simulink model "QArm_Test_2"  (R2021a)
settings: Solver=ode4  StartTime=0.0  StopTime=inf  FixedStep=1/500  RelTol=1e-3  EnableMultiTasking=on
InitFcn:
  | home = [0.45; 0; 0.49];
  | A = [0.45; 0; 0.49];
  | B = [ 0.35; -0.35; 0.59];
  | C = [ 0.35; -0.35; 0.39];
  | D = [ 0.35;  0.35; 0.39];
  | E = [ 0.35;  0.35; 0.59];
  | 
  | pick_high = [0.00; -0.45; 0.15];
  | pick = [0.00; -0.45; 0.03];
  | place = [0.00; 0.45; 0.15];
  | 
  | waypoints = ...
  | [B, B, C, D, D, E]' ;
undefined symbols (not defined in the file): HIL, qc_get_step_size
libraries: quarc_library x16, simulink x3
settings Model: SimulationMode=external  ExtModeTrigDuration=10000  Creator=fvranes  LastModifiedBy=mbohra
settings SolverCC: AlgebraicLoopSolver=TrustRegion  PositivePriorityOrder=on
settings DataIOCC: SaveOutput=off  SignalLogging=off  DSMLogging=off  SaveTime=off  ReturnWorkspaceOutputs=off
settings DebuggingCC: SFMachineParentedDataDiag=warning  ArithmeticOperatorsInVariantConditions=warning
settings SFSimCC: SimUseLocalCustomCode=off  CustomCodeUndefinedFunction=UseInterfaceOnly
settings RTWCC: Description=QUARC Win64 Target Using Toolchain  SystemTargetFile=quarc_win64.tlc  TemplateMakefile=quarc_default_tmf  RTWUseLocalCustomCode=off  Toolchain=QUARC win64 | nmake (64-bit Windows)  BuildConfiguration=Faster Runs
settings CodeAppCC: StateflowObjectComments=on
settings STFCustomTargetCC: TargetLangStandard=C99 (ISO)  ConcurrentExecutionCompliant=on  SystemTargetFile=quarc_win64.tlc
settings GRTTargetCC: ParMdlRefBuildCompliant=off  CompOptLevelCompliant=off  CombineOutputUpdateFcns=off  MatFileLogging=off  CPPClassGenCompliant=off  GRTInterface=on  ExtMode=on  ExtModeMexFile=quarc_comm
settings ConfigComp: CovMetricSettings=dswe

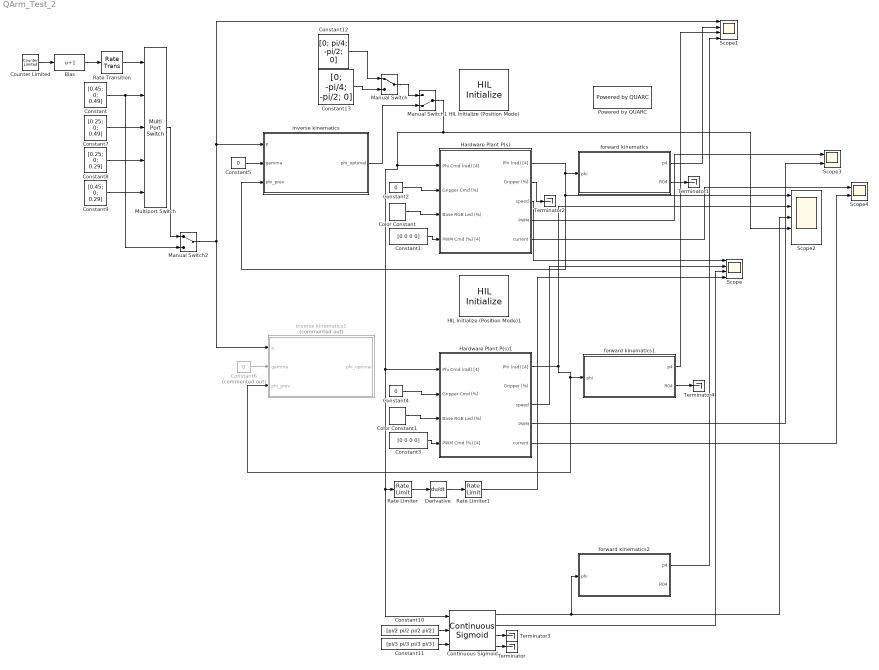
== system QArm_Test_2 ==
  Bias : Bias  Bias=1
  Color Constant : quarc_library/Sources/Signals/Color Constant  color=[0.71765 0.27451 1]
      settings: SourceProductName=QUARC Targets
  Color Constant1 : quarc_library/Sources/Signals/Color Constant  color=[0.71765 0.27451 1]
      settings: SourceProductName=QUARC Targets
  Constant : Constant  Value=[0.45; 0; 0.49]  VectorParams1D=off
  Constant1 : Constant  Value=[0 0 0 0]
  Constant10 : Constant  Value=[pi/2 pi/2 pi/2 pi/2]
  Constant11 : Constant  Value=[pi/3 pi/3 pi/3 pi/3]
  Constant12 : Constant  Value=[0; pi/4; -pi/2; 0]  VectorParams1D=off
  Constant13 : Constant  Value=[0; -pi/4; -pi/2; 0]  VectorParams1D=off
  Constant2 : Constant  Value=0
  Constant3 : Constant  Value=[0 0 0 0]
  Constant4 : Constant  Value=0
  Constant5 : Constant  Value=0
  Constant6 : Constant  Commented=on  Value=0
  Constant7 : Constant  Value=[0.25; 0; 0.49]  VectorParams1D=off
  Constant8 : Constant  Value=[0.25; 0; 0.29]  VectorParams1D=off
  Constant9 : Constant  Value=[0.45; 0; 0.29]  VectorParams1D=off
  Continuous Sigmoid : quarc_library/Sources/Sigmoids/Continuous Sigmoid  params_source=External (input ports)  max_velocity=10  max_acceleration=10  initial_position=0  initial_velocity=0  hold_off=qc_get_step_size  input_sample_time=qc_get_step_size  output_sample_time=qc_get_step_size
      settings: SourceProductName=QUARC Targets
  Counter Limited : simulink/Sources/Counter Limited  uplimit=3  tsamp=4
  Derivative : Derivative
  HIL Initialize (Position Mode) : quarc_library/Data Acquisition/Generic/Configuration/HIL Initialize  Priority=2  object_name=HIL-1  board_type=qarm_usb  board_number=0  board_options=j0_mode=0;j1_mode=0;j2_mode=0;j3_mode=0;gripper_mode=0;j0_profile_config=0;j0_profile_velocity=1.5708;j0_profile_acceleration=1.0472;j1_profile_config=0;j1_profile_velocity=1.5708;j1_profile_acceleration=1.0472;j2_profile_config=0;j2_profile_velocity=1.5708;j2_profile_acceleration=1.0472;j3_profile_config=0;j3_profile_velocity=1.5708;j3_profile_acceleration=1.0472;  exclusive=off  active=on  hardware_clocks=[0]  clock_modes=[]  initial_clock_frequencies=[]  set_clock_params_at_start=off  set_clock_params_at_switch_in=off  set_clock_frequencies_at_start=off  set_clock_frequencies_at_switch_in=off  analog_input_channels=[5:9]  analog_input_configurations=[]  analog_input_maximums=[]  analog_input_minimums=[]  set_analog_input_params_at_start=off  set_analog_input_params_at_switch_in=off  analog_output_channels=[]  analog_output_maximums=inf  analog_output_minimums=-inf  initial_analog_outputs=[0]  final_analog_outputs=[0]  watchdog_analog_outputs=[]  set_analog_output_params_at_start=off  set_analog_output_params_at_switch_in=off  set_analog_outputs_at_start=off  set_analog_outputs_at_switch_in=off  set_analog_outputs_at_terminate=off  set_analog_outputs_at_switch_out=off  set_analog_outputs_on_watchdog=off  digital_input_channels=[]  digital_output_channels=[]  digital_output_configuration=[]  initial_digital_outputs=[0]  final_digital_outputs=[0]  watchdog_digital_outputs=[0]  set_digital_output_params_at_start=off  set_digital_output_params_at_switch_in=off  set_digital_outputs_at_start=off  set_digital_outputs_at_switch_in=off  set_digital_outputs_at_terminate=off  set_digital_outputs_at_switch_out=off  set_digital_outputs_on_watchdog=off  encoder_channels=[]  quadrature=[]  encoder_filter_frequency=[]  initial_encoder_counts=[]  set_encoder_params_at_start=off  set_encoder_params_at_switch_in=off  set_encoder_counts_at_start=off  set_encoder_counts_at_switch_in=off  pwm_channels=[]  pwm_modes=[]  pwm_frequency=[]  pwm_configuration=[]  pwm_alignment=[]  pwm_polarity=[]  pwm_leading_deadband=[]  pwm_trailing_deadband=[]  initial_pwm_outputs=[]  final_pwm_outputs=[]  watchdog_pwm_outputs=[]  set_pwm_params_at_start=off  set_pwm_params_at_switch_in=off  set_pwm_outputs_at_start=off  set_pwm_outputs_at_switch_in=off  set_pwm_outputs_at_terminate=off  set_pwm_outputs_at_switch_out=off  set_pwm_outputs_on_watchdog=off  other_output_channels=[11005:11008]  initial_other_outputs=[0 1 0 1]  final_other_outputs=[1 0 0 0]  watchdog_other_outputs=[0 0 1 0]  set_other_outputs_at_start=on  set_other_outputs_at_switch_in=off  set_other_outputs_at_terminate=on  set_other_outputs_at_switch_out=off  set_other_outputs_on_watchdog=off
  HIL Initialize (Position Mode)1 : quarc_library/Data Acquisition/Generic/Configuration/HIL Initialize  Priority=2  object_name=HIL-2  board_type=qarm_usb  board_number=0@tcpip://localhost:18900  board_options=j0_mode=0;j1_mode=0;j2_mode=0;j3_mode=0;gripper_mode=0;j0_profile_config=0;j0_profile_velocity=1.5708;j0_profile_acceleration=1.0472;j1_profile_config=0;j1_profile_velocity=1.5708;j1_profile_acceleration=1.0472;j2_profile_config=0;j2_profile_velocity=1.5708;j2_profile_acceleration=1.0472;j3_profile_config=0;j3_profile_velocity=1.5708;j3_profile_acceleration=1.0472;  exclusive=off  active=on  hardware_clocks=[0]  clock_modes=[]  initial_clock_frequencies=[]  set_clock_params_at_start=off  set_clock_params_at_switch_in=off  set_clock_frequencies_at_start=off  set_clock_frequencies_at_switch_in=off  analog_input_channels=[5:9]  analog_input_configurations=[]  analog_input_maximums=[]  analog_input_minimums=[]  set_analog_input_params_at_start=off  set_analog_input_params_at_switch_in=off  analog_output_channels=[]  analog_output_maximums=inf  analog_output_minimums=-inf  initial_analog_outputs=[0]  final_analog_outputs=[0]  watchdog_analog_outputs=[]  set_analog_output_params_at_start=off  set_analog_output_params_at_switch_in=off  set_analog_outputs_at_start=off  set_analog_outputs_at_switch_in=off  set_analog_outputs_at_terminate=off  set_analog_outputs_at_switch_out=off  set_analog_outputs_on_watchdog=off  digital_input_channels=[]  digital_output_channels=[]  digital_output_configuration=[]  initial_digital_outputs=[0]  final_digital_outputs=[0]  watchdog_digital_outputs=[0]  set_digital_output_params_at_start=off  set_digital_output_params_at_switch_in=off  set_digital_outputs_at_start=off  set_digital_outputs_at_switch_in=off  set_digital_outputs_at_terminate=off  set_digital_outputs_at_switch_out=off  set_digital_outputs_on_watchdog=off  encoder_channels=[]  quadrature=[]  encoder_filter_frequency=[]  initial_encoder_counts=[]  set_encoder_params_at_start=off  set_encoder_params_at_switch_in=off  set_encoder_counts_at_start=off  set_encoder_counts_at_switch_in=off  pwm_channels=[]  pwm_modes=[]  pwm_frequency=[]  pwm_configuration=[]  pwm_alignment=[]  pwm_polarity=[]  pwm_leading_deadband=[]  pwm_trailing_deadband=[]  initial_pwm_outputs=[]  final_pwm_outputs=[]  watchdog_pwm_outputs=[]  set_pwm_params_at_start=off  set_pwm_params_at_switch_in=off  set_pwm_outputs_at_start=off  set_pwm_outputs_at_switch_in=off  set_pwm_outputs_at_terminate=off  set_pwm_outputs_at_switch_out=off  set_pwm_outputs_on_watchdog=off  other_output_channels=[11005:11008]  initial_other_outputs=[0 1 0 1]  final_other_outputs=[1 0 0 0]  watchdog_other_outputs=[0 0 1 0]  set_other_outputs_at_start=on  set_other_outputs_at_switch_in=off  set_other_outputs_at_terminate=on  set_other_outputs_at_switch_out=off  set_other_outputs_on_watchdog=off
  Hardware Plant P(s) : Subsystem
  Hardware Plant P(s)1 : Subsystem
  Manual Switch : ManualSwitch
  Manual Switch1 : ManualSwitch  CurrentSetting=0
  Manual Switch2 : ManualSwitch
  Multiport Switch : MultiPortSwitch  Inputs=4
  Powered by QUARC : quarc_library/Logos/Powered by QUARC
  Rate Limiter : RateLimiter  RisingSlewLimit=pi/2  FallingSlewLimit=-pi/2  SampleTimeMode=inherited
  Rate Limiter1 : RateLimiter  RisingSlewLimit=pi/3  FallingSlewLimit=-pi/3  SampleTimeMode=inherited
  Rate Transition : RateTransition
  Scope : Scope  NumInputPorts=4
  Scope1 : Scope  NumInputPorts=4
  Scope2 : Scope  NumInputPorts=5
  Scope3 : Scope  NumInputPorts=2
  Scope4 : Scope  NumInputPorts=2
  Terminator{,1..4} (5 alike) : Terminator
  forward kinematics : MATLAB Function  TreatAsAtomicUnit=on
  forward kinematics1 : MATLAB Function  TreatAsAtomicUnit=on
  forward kinematics2 : MATLAB Function  TreatAsAtomicUnit=on
  inverse kinematics : MATLAB Function  TreatAsAtomicUnit=on
  inverse kinematics1 : MATLAB Function  Commented=on  TreatAsAtomicUnit=on
  wires:
  Hardware Plant P(s)/2(Gripper (%)) -> Terminator2/1
  Hardware Plant P(s)/1(Phi (rad) [4]) -> inverse kinematics/3(phi_prev), Scope2/1, forward kinematics/1(phi)
  Color Constant/1 -> Hardware Plant P(s)/3(Base RGB Led (%))
  Constant1/1 -> Hardware Plant P(s)/4(PWM Cmd (%) [4])
  Constant5/1 -> inverse kinematics/2(gamma)
  Manual Switch1/1 -> Continuous Sigmoid/1, Rate Limiter/1, Hardware Plant P(s)1/1(Phi Cmd (rad) [4]), Hardware Plant P(s)/1(Phi Cmd (rad) [4]), Scope2/4
  Constant2/1 -> Hardware Plant P(s)/2(Gripper Cmd (%))
  forward kinematics/1(p4) -> Scope1/2
  forward kinematics/2(R04) -> Terminator1/1
  Constant4/1 -> Hardware Plant P(s)1/2(Gripper Cmd (%))
  Color Constant1/1 -> Hardware Plant P(s)1/3(Base RGB Led (%))
  Constant3/1 -> Hardware Plant P(s)1/4(PWM Cmd (%) [4])
  Manual Switch2/1 -> Scope1/1, inverse kinematics/1(p), inverse kinematics1/1(p)
  Constant6/1 -> inverse kinematics1/2(gamma)
  forward kinematics1/2(R04) -> Terminator4/1
  forward kinematics1/1(p4) -> Scope1/3
  Hardware Plant P(s)1/1(Phi (rad) [4]) -> inverse kinematics1/3(phi_prev), forward kinematics1/1(phi), Scope2/2
  Hardware Plant P(s)/3(speed) -> Scope/1
  Hardware Plant P(s)1/3(speed) -> Scope/2
  Constant/1 -> Manual Switch2/2, Multiport Switch/2
  Constant7/1 -> Multiport Switch/3
  Constant8/1 -> Multiport Switch/4
  Constant9/1 -> Multiport Switch/5
  Bias/1 -> Rate Transition/1
  Counter Limited/1 -> Bias/1
  Rate Transition/1 -> Multiport Switch/1
  Continuous Sigmoid/3 -> Terminator3/1
  Continuous Sigmoid/4 -> Terminator/1
  Constant11/1 -> Continuous Sigmoid/3
  Constant10/1 -> Continuous Sigmoid/2
  Continuous Sigmoid/1 -> forward kinematics2/1(phi), Scope2/3
  Continuous Sigmoid/2 -> Scope/3
  forward kinematics2/1(p4) -> Scope1/4
  Constant13/1 -> Manual Switch/2
  Constant12/1 -> Manual Switch/1
  Manual Switch/1 -> Manual Switch1/1
  inverse kinematics/1(phi_optimal) -> Manual Switch1/2
  Multiport Switch/1 -> Manual Switch2/1
  Rate Limiter/1 -> Derivative/1
  Derivative/1 -> Rate Limiter1/1
  Rate Limiter1/1 -> Scope/4
  Hardware Plant P(s)/4(PWM) -> Scope3/1
  Hardware Plant P(s)1/4(PWM) -> Scope3/2
  Hardware Plant P(s)/5(current) -> Scope4/1
  Hardware Plant P(s)1/5(current) -> Scope4/2

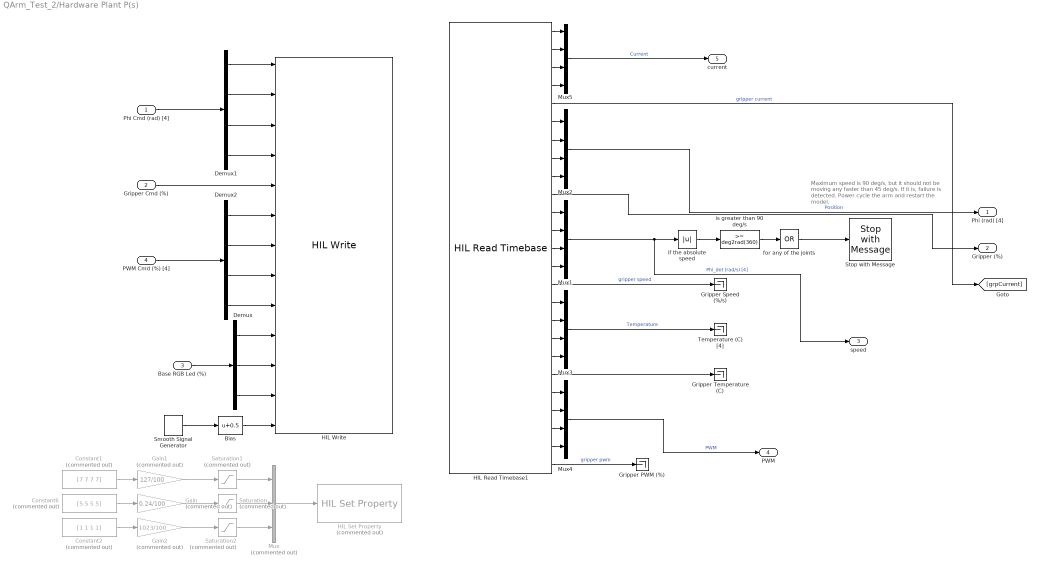
== system QArm_Test_2/Hardware Plant P(s) ==
  note: Maximum speed is 90 deg/s, but it should not
      | be moving any faster than 45 deg/s. If it is,
      | failure is detected. Power cycle the arm and
      | restart the model.
  Phi Cmd (rad) [4] : Inport
  Gripper Cmd (%) : Inport  Port=2
  Base RGB Led (%) : Inport  Port=3
  PWM Cmd (%) [4] : Inport  Port=4
  Bias : Bias  Bias=0.5
  Constant1 : Constant  Commented=on  Value=[7 7 7 7]
  Constant2 : Constant  Commented=on  Value=[1 1 1 1]
  Constant6 : Constant  Commented=on  Value=[5 5 5 5]
  Demux : Demux  Outputs=3
  Demux1 : Demux
  Demux2 : Demux
  Gain : Gain  Commented=on  Gain=0.24/100
  Gain1 : Gain  Commented=on  Gain=127/100
  Gain2 : Gain  Commented=on  Gain=1023/100
  Gripper PWM (%) : Terminator
  Gripper Speed (%/s) : Terminator
  Gripper Temperature (C) : Terminator
  HIL Read Timebase1 : quarc_library/Data Acquisition/Generic/Timebases/HIL Read Timebase  object_name=HIL-1  clock=0  analog_channels=[5:9]  encoder_channels=[]  digital_channels=[]  other_channels=[1000:1004 3000:3004 10000:10004 11000:11004]  active=on  vector_output=off  data_type_mode=Inherit via back propagation  encoder_data_type=double  digital_data_type=boolean  overflow_mode=Error on overflow  samples_in_buffer=max(ceil(1/qc_get_step_size), 1)
  HIL Set Property : quarc_library/Data Acquisition/Generic/Configuration/HIL Set Property  Commented=on  object_name=HIL-1  property_type=2  property_codes=[128:131, 133:136, 138:141]  property_source=2  property_value_num=0  set_at_start=on  sample_time=-1  active=off
      settings: AttributesFormatString=(%<object_name>)  SourceProductName=QUARC Targets
  HIL Write : quarc_library/Data Acquisition/Generic/Immediate I//O/HIL Write  object_name=HIL-1  analog_channels=[]  pwm_channels=[]  digital_channels=[]  other_channels=[1000:1004 11000:11003 11005:11008]  sample_time=-1  active=on  vector_input=off
  Mux : Mux  Commented=on  Inputs=3
  Mux{1..5} (5 alike) : Mux
  Saturation : Saturate  Commented=on  UpperLimit=0.24  LowerLimit=0
  Saturation1 : Saturate  Commented=on  UpperLimit=127  LowerLimit=0
  Saturation2 : Saturate  Commented=on  UpperLimit=1023  LowerLimit=0
  Smooth Signal Generator : quarc_library/Sources/Signals/Smooth Signal Generator  signal_type=Sine  source=Internal (dialog parameters)  amplitude=0.5  frequency=0.5  initial_phase=0  sample_time=qc_get_step_size  output_cos=off
      settings: SourceProductName=QUARC Targets
  Stop with Message : quarc_library/Sinks/Error Handling/Stop with Message  message_type=Fixed error message  message_icon=Error  message=Arm moving close to maximum speed.
  Temperature (C) [4] : Terminator
  for any of the joints : Logic  Operator=OR  Inputs=1  IconShape=distinctive  AllPortsSameDT=off  OutDataTypeStr=boolean
  if the absolute speed : Abs
  is greater than 90 deg/s : simulink/Logic and Bit Operations/Compare To Constant  relop=>=  const=deg2rad(360)  OutDataTypeStr=boolean
  Phi (rad) [4] : Outport  VectorParamsAs1DForOutWhenUnconnected=off
  Gripper (%) : Outport  Port=2  VectorParamsAs1DForOutWhenUnconnected=off
  speed : Outport  Port=3  VectorParamsAs1DForOutWhenUnconnected=off
  PWM : Outport  Port=4  VectorParamsAs1DForOutWhenUnconnected=off
  current : Outport  Port=5  VectorParamsAs1DForOutWhenUnconnected=off
  wires:
  HIL Read Timebase1/10 -> Gripper (%)/1
  Constant6/1 -> Gain/1
  Saturation/1 -> Mux/2
  Gain/1 -> Saturation/1
  Mux/1 -> HIL Set Property/1
  Gain1/1 -> Saturation1/1
  Constant1/1 -> Gain1/1
  Constant2/1 -> Gain2/1
  Gain2/1 -> Saturation2/1
  Saturation2/1 -> Mux/3
  Saturation1/1 -> Mux/1
  Demux1/4 -> HIL Write/4
  Base RGB Led (%)/1 -> Demux/1
  Demux/2 -> HIL Write/11
  Demux/1 -> HIL Write/10
  Demux1/2 -> HIL Write/2
  Gripper Cmd (%)/1 -> HIL Write/5
  Bias/1 -> HIL Write/13
  Phi Cmd (rad) [4]/1 -> Demux1/1
  Smooth Signal Generator/1 -> Bias/1
  Demux/3 -> HIL Write/12
  Demux1/3 -> HIL Write/3
  PWM Cmd (%) [4]/1 -> Demux2/1
  Demux2/2 -> HIL Write/7
  Demux2/1 -> HIL Write/6
  Demux1/1 -> HIL Write/1
  Demux2/4 -> HIL Write/9
  Demux2/3 -> HIL Write/8
  for any of the joints/1 -> Stop with Message/1
  is greater than 90 deg/s/1 -> for any of the joints/1
  if the absolute speed/1 -> is greater than 90 deg/s/1
  HIL Read Timebase1/16 -> Mux3/1
  HIL Read Timebase1/12 -> Mux1/2
  HIL Read Timebase1/4 -> Mux5/4
  HIL Read Timebase1/5 -> [grpCurrent]  "gripper current"
  HIL Read Timebase1/11 -> Mux1/1
  HIL Read Timebase1/14 -> Mux1/4
  HIL Read Timebase1/6 -> Mux2/1
  HIL Read Timebase1/19 -> Mux3/4
  HIL Read Timebase1/8 -> Mux2/3
  Mux5/1 -> current/1  "Current"
  HIL Read Timebase1/7 -> Mux2/2
  HIL Read Timebase1/24 -> Mux4/4
  HIL Read Timebase1/1 -> Mux5/1
  HIL Read Timebase1/2 -> Mux5/2
  HIL Read Timebase1/21 -> Mux4/1
  HIL Read Timebase1/20 -> Gripper Temperature (C)/1
  HIL Read Timebase1/22 -> Mux4/2
  HIL Read Timebase1/17 -> Mux3/2
  HIL Read Timebase1/18 -> Mux3/3
  Mux4/1 -> PWM/1  "PWM"
  HIL Read Timebase1/13 -> Mux1/3
  HIL Read Timebase1/23 -> Mux4/3
  HIL Read Timebase1/3 -> Mux5/3
  HIL Read Timebase1/25 -> Gripper PWM (%)/1  "gripper pwm"
  Mux3/1 -> Temperature (C) [4]/1  "Temperature"
  HIL Read Timebase1/9 -> Mux2/4
  Mux2/1 -> Phi (rad) [4]/1  "Position"
  Mux1/1 -> speed/1, if the absolute speed/1  "Phi_dot (rad/s) [4]"
  HIL Read Timebase1/15 -> Gripper Speed (%/s)/1  "gripper speed"

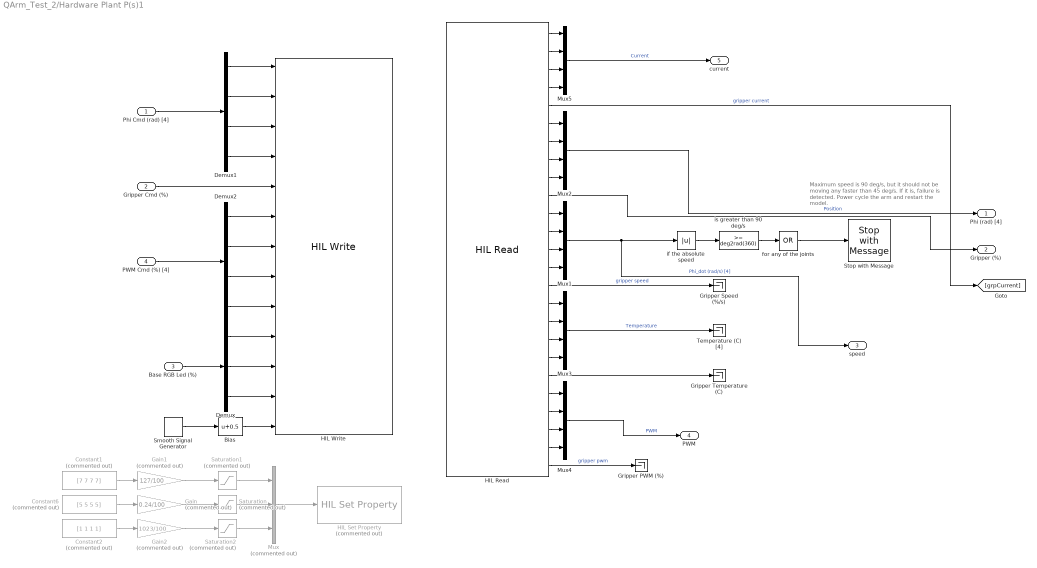
== system QArm_Test_2/Hardware Plant P(s)1 ==
  note: Maximum speed is 90 deg/s, but it should not
      | be moving any faster than 45 deg/s. If it is,
      | failure is detected. Power cycle the arm and
      | restart the model.
  Phi Cmd (rad) [4] : Inport
  Gripper Cmd (%) : Inport  Port=2
  Base RGB Led (%) : Inport  Port=3
  PWM Cmd (%) [4] : Inport  Port=4
  Bias : Bias  Bias=0.5
  Constant1 : Constant  Commented=on  Value=[7 7 7 7]
  Constant2 : Constant  Commented=on  Value=[1 1 1 1]
  Constant6 : Constant  Commented=on  Value=[5 5 5 5]
  Demux : Demux  Outputs=3
  Demux1 : Demux
  Demux2 : Demux
  Gain : Gain  Commented=on  Gain=0.24/100
  Gain1 : Gain  Commented=on  Gain=127/100
  Gain2 : Gain  Commented=on  Gain=1023/100
  Gripper PWM (%) : Terminator
  Gripper Speed (%/s) : Terminator
  Gripper Temperature (C) : Terminator
  HIL Read : quarc_library/Data Acquisition/Generic/Immediate I//O/HIL Read  object_name=HIL-2  analog_channels=[5:9]  encoder_channels=[]  digital_channels=[]  other_channels=[1000:1004 3000:3004 10000:10004 11000:11004]  sample_time=qc_get_step_size  active=on  vector_output=off  data_type_mode=Inherit via back propagation  encoder_data_type=double  digital_data_type=boolean
  HIL Set Property : quarc_library/Data Acquisition/Generic/Configuration/HIL Set Property  Commented=on  object_name=HIL-2  property_type=2  property_codes=[128:131, 133:136, 138:141]  property_source=2  property_value_num=0  set_at_start=on  sample_time=-1  active=off
      settings: AttributesFormatString=(%<object_name>)  SourceProductName=QUARC Targets
  HIL Write : quarc_library/Data Acquisition/Generic/Immediate I//O/HIL Write  object_name=HIL-2  analog_channels=[]  pwm_channels=[]  digital_channels=[]  other_channels=[1000:1004 11000:11003 11005:11008]  sample_time=-1  active=on  vector_input=off
  Mux : Mux  Commented=on  Inputs=3
  Mux{1..5} (5 alike) : Mux
  Saturation : Saturate  Commented=on  UpperLimit=0.24  LowerLimit=0
  Saturation1 : Saturate  Commented=on  UpperLimit=127  LowerLimit=0
  Saturation2 : Saturate  Commented=on  UpperLimit=1023  LowerLimit=0
  Smooth Signal Generator : quarc_library/Sources/Signals/Smooth Signal Generator  signal_type=Sine  source=Internal (dialog parameters)  amplitude=0.5  frequency=0.5  initial_phase=0  sample_time=qc_get_step_size  output_cos=off
      settings: SourceProductName=QUARC Targets
  Stop with Message : quarc_library/Sinks/Error Handling/Stop with Message  message_type=Fixed error message  message_icon=Error  message=Arm moving close to maximum speed.
  Temperature (C) [4] : Terminator
  for any of the joints : Logic  Operator=OR  Inputs=1  IconShape=distinctive  AllPortsSameDT=off  OutDataTypeStr=boolean
  if the absolute speed : Abs
  is greater than 90 deg/s : simulink/Logic and Bit Operations/Compare To Constant  relop=>=  const=deg2rad(360)  OutDataTypeStr=boolean
  Phi (rad) [4] : Outport  VectorParamsAs1DForOutWhenUnconnected=off
  Gripper (%) : Outport  Port=2  VectorParamsAs1DForOutWhenUnconnected=off
  speed : Outport  Port=3  VectorParamsAs1DForOutWhenUnconnected=off
  PWM : Outport  Port=4  VectorParamsAs1DForOutWhenUnconnected=off
  current : Outport  Port=5  VectorParamsAs1DForOutWhenUnconnected=off
  wires:
  HIL Read/15 -> Gripper Speed (%/s)/1  "gripper speed"
  Mux2/1 -> Phi (rad) [4]/1  "Position"
  HIL Read/9 -> Mux2/4
  Mux3/1 -> Temperature (C) [4]/1  "Temperature"
  HIL Read/25 -> Gripper PWM (%)/1  "gripper pwm"
  HIL Read/3 -> Mux5/3
  HIL Read/23 -> Mux4/3
  HIL Read/13 -> Mux1/3
  Mux4/1 -> PWM/1  "PWM"
  HIL Read/18 -> Mux3/3
  HIL Read/17 -> Mux3/2
  HIL Read/22 -> Mux4/2
  HIL Read/20 -> Gripper Temperature (C)/1
  HIL Read/21 -> Mux4/1
  HIL Read/2 -> Mux5/2
  HIL Read/1 -> Mux5/1
  HIL Read/24 -> Mux4/4
  HIL Read/7 -> Mux2/2
  Mux5/1 -> current/1  "Current"
  HIL Read/8 -> Mux2/3
  HIL Read/19 -> Mux3/4
  HIL Read/6 -> Mux2/1
  HIL Read/14 -> Mux1/4
  HIL Read/11 -> Mux1/1
  HIL Read/5 -> [grpCurrent]  "gripper current"
  HIL Read/4 -> Mux5/4
  HIL Read/12 -> Mux1/2
  HIL Read/16 -> Mux3/1
  if the absolute speed/1 -> is greater than 90 deg/s/1
  is greater than 90 deg/s/1 -> for any of the joints/1
  for any of the joints/1 -> Stop with Message/1
  Demux2/3 -> HIL Write/8
  Demux2/4 -> HIL Write/9
  Demux1/1 -> HIL Write/1
  Demux2/1 -> HIL Write/6
  Demux2/2 -> HIL Write/7
  PWM Cmd (%) [4]/1 -> Demux2/1
  Demux1/3 -> HIL Write/3
  Demux/3 -> HIL Write/12
  Smooth Signal Generator/1 -> Bias/1
  Phi Cmd (rad) [4]/1 -> Demux1/1
  Bias/1 -> HIL Write/13
  Gripper Cmd (%)/1 -> HIL Write/5
  Demux1/2 -> HIL Write/2
  Demux/1 -> HIL Write/10
  Demux/2 -> HIL Write/11
  Base RGB Led (%)/1 -> Demux/1
  Demux1/4 -> HIL Write/4
  Saturation1/1 -> Mux/1
  Saturation2/1 -> Mux/3
  Gain2/1 -> Saturation2/1
  Constant2/1 -> Gain2/1
  Constant1/1 -> Gain1/1
  Gain1/1 -> Saturation1/1
  Mux/1 -> HIL Set Property/1
  Gain/1 -> Saturation/1
  Saturation/1 -> Mux/2
  Constant6/1 -> Gain/1
  HIL Read/10 -> Gripper (%)/1
  Mux1/1 -> speed/1, if the absolute speed/1  "Phi_dot (rad/s) [4]"

== matlab function QArm_Test_2/inverse kinematics1 ==
  data: p input; gamma input; phi_optimal output; phi_prev input
function phi_optimal = qarmInverseKinematics(p, gamma, phi_prev)

%% QUANSER_ARM_IPK
% v 4.0 - 4th June 2020

% REFERENCE: 
% Chapter 4. Inverse Kinematics
% Robot Dynamics and Control 
% Spong, Vidyasagar
% 1989

% INPUTS:
% p        : end-effector position vector expressed in base frame {0}
% gamma    : wrist rotation angle gamma

% OUTPUTS:
% phi_optimal : Best solution depending on phi_prev
% phi         : All four Inverse Kinematics solutions as a 4x4 matrix. 
%               Each col is a solution.

%% Manipulator parameters:
L1 = 0.1400;
L2 = 0.3500;
L3 = 0.0500;
L4 = 0.2500;
L5 = 0.1500;
beta = atan(L3/L2);

%% Alternate parameters
lambda1 = L1;
lambda2 = sqrt(L2^2 + L3^2);
lambda3 = L4 + L5;

%% Initialization
theta   = zeros(4, 4);
phi = zeros(4, 4);

%% Joint angle 2 and 3: 
% Equations:
    % lambda2 cos(theta2) + (-lambda3) sin(theta2 + theta3) = sqrt(x^2 + y^2)
    %   A     cos( 2    ) +     C      sin(   2   +    3  ) =    D
    
    % lambda2 sin(theta2) - (-lambda3) cos(theta2 + theta3) = lambda1 - z
    %   A     sin( 2    ) -     C      cos(   2   +    3  ) =    H

% Solution:
    A = lambda2;
    C = -lambda3;
    H =  lambda1 - p(3);
    D1 = -sqrt(p(1)^2 + p(2)^2);
    D2 = sqrt(p(1)^2 + p(2)^2);
    F = (D1^2 + H^2 - A^2 - C^2)/(2*A);

    theta(3,1) = 2*atan2( C + sqrt(C^2 - F^2) , F );
	theta(3,2) = 2*atan2( C - sqrt(C^2 - F^2) , F );
    theta(3,3) = 2*atan2( C + sqrt(C^2 - F^2) , F );
	theta(3,4) = 2*atan2( C - sqrt(C^2 - F^2) , F );

    M = A + C*sin(theta(3,1));
    N = -C*cos(theta(3,1));
    cos_term = (D1*M + H*N)/(M^2 + N^2);
    sin_term = (H - N*cos_term)/(M);
    theta(2,1) = atan2(sin_term, cos_term);

    M = A + C*sin(theta(3,2));
    N = -C*cos(theta(3,2));
    cos_term = (D1*M + H*N)/(M^2 + N^2);
    sin_term = (H - N*cos_term)/(M);
    theta(2,2) = atan2(sin_term, cos_term);

    M = A + C*sin(theta(3,3));
    N = -C*cos(theta(3,3));
    cos_term = (D2*M + H*N)/(M^2 + N^2);
    sin_term = (H - N*cos_term)/(M);
    theta(2,3) = atan2(sin_term, cos_term);

    M = A + C*sin(theta(3,4));
    N = -C*cos(theta(3,4));
    cos_term = (D2*M + H*N)/(M^2 + N^2);
    sin_term = (H - N*cos_term)/(M);
    theta(2,4) = atan2(sin_term, cos_term);


%% Joint angle 1:
% Equation:
    % y / x = tan(theta1);

% Solution
    theta(1,1) = atan2( p(2)/( lambda2 * cos( theta(2,1) ) - lambda3 * sin( theta(2,1) + theta(3,1) ) ) , p(1)/(  lambda2 * cos( theta(2,1) ) - lambda3 * sin( theta(2,1) + theta(3,1) )  ) );
    theta(1,2) = atan2( p(2)/( lambda2 * cos( theta(2,2) ) - lambda3 * sin( theta(2,2) + theta(3,2) ) ) , p(1)/(  lambda2 * cos( theta(2,2) ) - lambda3 * sin( theta(2,2) + theta(3,2) )  ) );
    theta(1,3) = atan2( p(2)/( lambda2 * cos( theta(2,3) ) - lambda3 * sin( theta(2,3) + theta(3,3) ) ) , p(1)/(  lambda2 * cos( theta(2,3) ) - lambda3 * sin( theta(2,3) + theta(3,3) )  ) );
    theta(1,4) = atan2( p(2)/( lambda2 * cos( theta(2,4) ) - lambda3 * sin( theta(2,4) + theta(3,4) ) ) , p(1)/(  lambda2 * cos( theta(2,4) ) - lambda3 * sin( theta(2,4) + theta(3,4) )  ) );
    
%% Remap theta back to phi
% phi(1) = theta(1);
% phi(2) = theta(2) - beta + pi/2;
% phi(3) = theta(3) + beta;
% phi(4) = theta(4);

phi(1,:) = theta(1,:);
phi(2,:) = theta(2,:) - beta + pi/2;
phi(3,:) = theta(3,:) + beta;
phi(4,:) = gamma;

phi = mod(phi + pi, 2*pi) - pi;

phi_optimal = phi(:,1);
if (norm(phi_optimal - phi_prev) > norm(phi(:,2) - phi_prev)) || (check_joint_limits(phi_optimal))
    phi_optimal = phi(:,2);
end
if (norm(phi_optimal - phi_prev) > norm(phi(:,3) - phi_prev)) || (check_joint_limits(phi_optimal))
    phi_optimal = phi(:,3);
end
if (norm(phi_optimal - phi_prev) > norm(phi(:,4) - phi_prev)) || (check_joint_limits(phi_optimal))
    phi_optimal = phi(:,4);
end
if (check_joint_limits(phi_optimal))
    phi_optimal = [0;0;0;0];
end

end

function flag = check_joint_limits(phi)
    flag = 0;
    if phi(1) > 170*pi/180 || phi(1) < -170*pi/180 ...
        || phi(2) > 80*pi/180 || phi(2) < -80*pi/180 ...
        || phi(3) > 75*pi/180 || phi(3) < -95*pi/180 ...
        || phi(4) > 160*pi/180 || phi(4) < -160*pi/180
    flag = 1;
    end
end

== matlab function QArm_Test_2/forward kinematics1 ==
  data: phi input; p4 output; R04 output
function [p4, R04] = qarmForwardKinematics(phi)

%% QUANSER_ARM_FPK
% v 4.0 - 4th June 2020

% REFERENCE: 
% Chapter 3. Forward Kinematics
% Robot Dynamics and Control 
% Spong, Vidyasagar
% 1989

% INPUTS:
% phi     : Alternate joint angles vector 4 x 1

% OUTPUTS:
% p4      : End-effector frame {4} position vector expressed in base frame {0}
% R04     : rotation matrix from end-effector frame {4} to base frame {0}

%% Manipulator parameters:
L1 = 0.1400;
L2 = 0.3500;
L3 = 0.0500;
L4 = 0.2500;
L5 = 0.1500;

%% Alternate parameters
l1 = L1;
l2 = sqrt(L2^2 + L3^2);
l3 = L4 + L5;
beta = atan(L3/L2);

%% From phi space to theta space 
theta = phi;
theta(1) = phi(1);
theta(2) = phi(2) + beta - pi/2;
theta(3) = phi(3) - beta;
theta(4) = phi(4);

%% Transformation matrices for all frames:

% T{i-1}{i} = quanser_arm_DH(  a, alpha,  d,     theta );
        T01 = quanser_arm_DH(  0, -pi/2, l1,  theta(1) );
        T12 = quanser_arm_DH( l2,     0,  0,  theta(2) );
        T23 = quanser_arm_DH(  0, -pi/2,  0,  theta(3) );
        T34 = quanser_arm_DH(  0,     0, l3,  theta(4) );

        T02 = T01*T12;
        T03 = T02*T23;
        T04 = T03*T34;

%% Position of end-effector Transformation

% Extract the Position vector 
% p1   = T01(1:3,4);
% p2   = T02(1:3,4);
% p3   = T03(1:3,4);
p4   = T04(1:3,4);

% Extract the Rotation matrix
% R01 = T01(1:3,1:3);
% R02 = T02(1:3,1:3);
% R03 = T03(1:3,1:3);
R04 = T04(1:3,1:3);

end

function T = quanser_arm_DH(a,alpha,d,theta)

%% QUANSER_ARM_DH
% v 1.0 - 26th March 2019

% REFERENCE: 
% Chapter 3. Forward and Inverse Kinematics
% Robot Modeling and Control 
% Spong, Hutchinson, Vidyasagar
% 2006

% INPUTS:
% a       :   translation  : along : x_{i}   : from : z_{i-1} : to : z_{i}
% alpha   :      rotation  : about : x_{i}   : from : z_{i-1} : to : z_{i}
% d       :   translation  : along : z_{i-1} : from : x_{i-1} : to : x_{i}
% theta   :      rotation  : about : z_{i-1} : from : x_{i-1} : to : x_{i}
% NOTE: Standard DH Parameters

% OUTPUTS:
% T       : transformation                   : from :     {i} : to : {i-1}

%%
% Rotation Transformation about z axis by theta
T_R_z = [cos(theta) -sin(theta) 0 0;
         sin(theta)  cos(theta) 0 0;
                  0           0 1 0;
                  0           0 0 1];
     
% Translation Transformation along z axis by d
T_T_z = [1 0 0 0;
         0 1 0 0;
         0 0 1 d;
         0 0 0 1];

% Translation Transformation along x axis by a
T_T_x = [1 0 0 a;
         0 1 0 0;
         0 0 1 0;
         0 0 0 1];

% Rotation Transformation about x axis by alpha
T_R_x = [1          0           0 0;
         0 cos(alpha) -sin(alpha) 0;
         0 sin(alpha)  cos(alpha) 0;
         0          0           0 1];

% For a transformation FROM frame {i} TO frame {i-1}: A
T = T_R_z*T_T_z*T_T_x*T_R_x;

end

== matlab function QArm_Test_2/forward kinematics ==
  data: phi input; p4 output; R04 output
function [p4, R04] = qarmForwardKinematics(phi)

%% QUANSER_ARM_FPK
% v 4.0 - 4th June 2020

% REFERENCE: 
% Chapter 3. Forward Kinematics
% Robot Dynamics and Control 
% Spong, Vidyasagar
% 1989

% INPUTS:
% phi     : Alternate joint angles vector 4 x 1

% OUTPUTS:
% p4      : End-effector frame {4} position vector expressed in base frame {0}
% R04     : rotation matrix from end-effector frame {4} to base frame {0}

%% Manipulator parameters:
L1 = 0.1400;
L2 = 0.3500;
L3 = 0.0500;
L4 = 0.2500;
L5 = 0.1500;

%% Alternate parameters
l1 = L1;
l2 = sqrt(L2^2 + L3^2);
l3 = L4 + L5;
beta = atan(L3/L2);

%% From phi space to theta space 
theta = phi;
theta(1) = phi(1);
theta(2) = phi(2) + beta - pi/2;
theta(3) = phi(3) - beta;
theta(4) = phi(4);

%% Transformation matrices for all frames:

% T{i-1}{i} = quanser_arm_DH(  a, alpha,  d,     theta );
        T01 = quanser_arm_DH(  0, -pi/2, l1,  theta(1) );
        T12 = quanser_arm_DH( l2,     0,  0,  theta(2) );
        T23 = quanser_arm_DH(  0, -pi/2,  0,  theta(3) );
        T34 = quanser_arm_DH(  0,     0, l3,  theta(4) );

        T02 = T01*T12;
        T03 = T02*T23;
        T04 = T03*T34;

%% Position of end-effector Transformation

% Extract the Position vector 
% p1   = T01(1:3,4);
% p2   = T02(1:3,4);
% p3   = T03(1:3,4);
p4   = T04(1:3,4);

% Extract the Rotation matrix
% R01 = T01(1:3,1:3);
% R02 = T02(1:3,1:3);
% R03 = T03(1:3,1:3);
R04 = T04(1:3,1:3);

end

function T = quanser_arm_DH(a,alpha,d,theta)

%% QUANSER_ARM_DH
% v 1.0 - 26th March 2019

% REFERENCE: 
% Chapter 3. Forward and Inverse Kinematics
% Robot Modeling and Control 
% Spong, Hutchinson, Vidyasagar
% 2006

% INPUTS:
% a       :   translation  : along : x_{i}   : from : z_{i-1} : to : z_{i}
% alpha   :      rotation  : about : x_{i}   : from : z_{i-1} : to : z_{i}
% d       :   translation  : along : z_{i-1} : from : x_{i-1} : to : x_{i}
% theta   :      rotation  : about : z_{i-1} : from : x_{i-1} : to : x_{i}
% NOTE: Standard DH Parameters

% OUTPUTS:
% T       : transformation                   : from :     {i} : to : {i-1}

%%
% Rotation Transformation about z axis by theta
T_R_z = [cos(theta) -sin(theta) 0 0;
         sin(theta)  cos(theta) 0 0;
                  0           0 1 0;
                  0           0 0 1];
     
% Translation Transformation along z axis by d
T_T_z = [1 0 0 0;
         0 1 0 0;
         0 0 1 d;
         0 0 0 1];

% Translation Transformation along x axis by a
T_T_x = [1 0 0 a;
         0 1 0 0;
         0 0 1 0;
         0 0 0 1];

% Rotation Transformation about x axis by alpha
T_R_x = [1          0           0 0;
         0 cos(alpha) -sin(alpha) 0;
         0 sin(alpha)  cos(alpha) 0;
         0          0           0 1];

% For a transformation FROM frame {i} TO frame {i-1}: A
T = T_R_z*T_T_z*T_T_x*T_R_x;

end

== matlab function QArm_Test_2/inverse kinematics ==
  data: p input; gamma input; phi_optimal output; phi_prev input
function phi_optimal = qarmInverseKinematics(p, gamma, phi_prev)

%% QUANSER_ARM_IPK
% v 4.0 - 4th June 2020

% REFERENCE: 
% Chapter 4. Inverse Kinematics
% Robot Dynamics and Control 
% Spong, Vidyasagar
% 1989

% INPUTS:
% p        : end-effector position vector expressed in base frame {0}
% gamma    : wrist rotation angle gamma

% OUTPUTS:
% phi_optimal : Best solution depending on phi_prev
% phi         : All four Inverse Kinematics solutions as a 4x4 matrix. 
%               Each col is a solution.

%% Manipulator parameters:
L1 = 0.1400;
L2 = 0.3500;
L3 = 0.0500;
L4 = 0.2500;
L5 = 0.1500;
beta = atan(L3/L2);

%% Alternate parameters
lambda1 = L1;
lambda2 = sqrt(L2^2 + L3^2);
lambda3 = L4 + L5;

%% Initialization
theta   = zeros(4, 4);
phi = zeros(4, 4);

%% Joint angle 2 and 3: 
% Equations:
    % lambda2 cos(theta2) + (-lambda3) sin(theta2 + theta3) = sqrt(x^2 + y^2)
    %   A     cos( 2    ) +     C      sin(   2   +    3  ) =    D
    
    % lambda2 sin(theta2) - (-lambda3) cos(theta2 + theta3) = lambda1 - z
    %   A     sin( 2    ) -     C      cos(   2   +    3  ) =    H

% Solution:
    A = lambda2;
    C = -lambda3;
    H =  lambda1 - p(3);
    D1 = -sqrt(p(1)^2 + p(2)^2);
    D2 = sqrt(p(1)^2 + p(2)^2);
    F = (D1^2 + H^2 - A^2 - C^2)/(2*A);

    theta(3,1) = 2*atan2( C + sqrt(C^2 - F^2) , F );
	theta(3,2) = 2*atan2( C - sqrt(C^2 - F^2) , F );
    theta(3,3) = 2*atan2( C + sqrt(C^2 - F^2) , F );
	theta(3,4) = 2*atan2( C - sqrt(C^2 - F^2) , F );

    M = A + C*sin(theta(3,1));
    N = -C*cos(theta(3,1));
    cos_term = (D1*M + H*N)/(M^2 + N^2);
    sin_term = (H - N*cos_term)/(M);
    theta(2,1) = atan2(sin_term, cos_term);

    M = A + C*sin(theta(3,2));
    N = -C*cos(theta(3,2));
    cos_term = (D1*M + H*N)/(M^2 + N^2);
    sin_term = (H - N*cos_term)/(M);
    theta(2,2) = atan2(sin_term, cos_term);

    M = A + C*sin(theta(3,3));
    N = -C*cos(theta(3,3));
    cos_term = (D2*M + H*N)/(M^2 + N^2);
    sin_term = (H - N*cos_term)/(M);
    theta(2,3) = atan2(sin_term, cos_term);

    M = A + C*sin(theta(3,4));
    N = -C*cos(theta(3,4));
    cos_term = (D2*M + H*N)/(M^2 + N^2);
    sin_term = (H - N*cos_term)/(M);
    theta(2,4) = atan2(sin_term, cos_term);


%% Joint angle 1:
% Equation:
    % y / x = tan(theta1);

% Solution
    theta(1,1) = atan2( p(2)/( lambda2 * cos( theta(2,1) ) - lambda3 * sin( theta(2,1) + theta(3,1) ) ) , p(1)/(  lambda2 * cos( theta(2,1) ) - lambda3 * sin( theta(2,1) + theta(3,1) )  ) );
    theta(1,2) = atan2( p(2)/( lambda2 * cos( theta(2,2) ) - lambda3 * sin( theta(2,2) + theta(3,2) ) ) , p(1)/(  lambda2 * cos( theta(2,2) ) - lambda3 * sin( theta(2,2) + theta(3,2) )  ) );
    theta(1,3) = atan2( p(2)/( lambda2 * cos( theta(2,3) ) - lambda3 * sin( theta(2,3) + theta(3,3) ) ) , p(1)/(  lambda2 * cos( theta(2,3) ) - lambda3 * sin( theta(2,3) + theta(3,3) )  ) );
    theta(1,4) = atan2( p(2)/( lambda2 * cos( theta(2,4) ) - lambda3 * sin( theta(2,4) + theta(3,4) ) ) , p(1)/(  lambda2 * cos( theta(2,4) ) - lambda3 * sin( theta(2,4) + theta(3,4) )  ) );
    
%% Remap theta back to phi
% phi(1) = theta(1);
% phi(2) = theta(2) - beta + pi/2;
% phi(3) = theta(3) + beta;
% phi(4) = theta(4);

phi(1,:) = theta(1,:);
phi(2,:) = theta(2,:) - beta + pi/2;
phi(3,:) = theta(3,:) + beta;
phi(4,:) = gamma;

phi = mod(phi + pi, 2*pi) - pi;

phi_optimal = phi(:,1);
if (norm(phi_optimal - phi_prev) > norm(phi(:,2) - phi_prev)) || (check_joint_limits(phi_optimal))
    phi_optimal = phi(:,2);
end
if (norm(phi_optimal - phi_prev) > norm(phi(:,3) - phi_prev)) || (check_joint_limits(phi_optimal))
    phi_optimal = phi(:,3);
end
if (norm(phi_optimal - phi_prev) > norm(phi(:,4) - phi_prev)) || (check_joint_limits(phi_optimal))
    phi_optimal = phi(:,4);
end
if (check_joint_limits(phi_optimal))
    phi_optimal = [0;0;0;0];
end

end

function flag = check_joint_limits(phi)
    flag = 0;
    if phi(1) > 170*pi/180 || phi(1) < -170*pi/180 ...
        || phi(2) > 80*pi/180 || phi(2) < -80*pi/180 ...
        || phi(3) > 75*pi/180 || phi(3) < -95*pi/180 ...
        || phi(4) > 160*pi/180 || phi(4) < -160*pi/180
    flag = 1;
    end
end

== matlab function QArm_Test_2/forward kinematics2 ==
  data: phi input; p4 output; R04 output
function [p4, R04] = qarmForwardKinematics(phi)

%% QUANSER_ARM_FPK
% v 4.0 - 4th June 2020

% REFERENCE: 
% Chapter 3. Forward Kinematics
% Robot Dynamics and Control 
% Spong, Vidyasagar
% 1989

% INPUTS:
% phi     : Alternate joint angles vector 4 x 1

% OUTPUTS:
% p4      : End-effector frame {4} position vector expressed in base frame {0}
% R04     : rotation matrix from end-effector frame {4} to base frame {0}

%% Manipulator parameters:
L1 = 0.1400;
L2 = 0.3500;
L3 = 0.0500;
L4 = 0.2500;
L5 = 0.1500;

%% Alternate parameters
l1 = L1;
l2 = sqrt(L2^2 + L3^2);
l3 = L4 + L5;
beta = atan(L3/L2);

%% From phi space to theta space 
theta = phi;
theta(1) = phi(1);
theta(2) = phi(2) + beta - pi/2;
theta(3) = phi(3) - beta;
theta(4) = phi(4);

%% Transformation matrices for all frames:

% T{i-1}{i} = quanser_arm_DH(  a, alpha,  d,     theta );
        T01 = quanser_arm_DH(  0, -pi/2, l1,  theta(1) );
        T12 = quanser_arm_DH( l2,     0,  0,  theta(2) );
        T23 = quanser_arm_DH(  0, -pi/2,  0,  theta(3) );
        T34 = quanser_arm_DH(  0,     0, l3,  theta(4) );

        T02 = T01*T12;
        T03 = T02*T23;
        T04 = T03*T34;

%% Position of end-effector Transformation

% Extract the Position vector 
% p1   = T01(1:3,4);
% p2   = T02(1:3,4);
% p3   = T03(1:3,4);
p4   = T04(1:3,4);

% Extract the Rotation matrix
% R01 = T01(1:3,1:3);
% R02 = T02(1:3,1:3);
% R03 = T03(1:3,1:3);
R04 = T04(1:3,1:3);

end

function T = quanser_arm_DH(a,alpha,d,theta)

%% QUANSER_ARM_DH
% v 1.0 - 26th March 2019

% REFERENCE: 
% Chapter 3. Forward and Inverse Kinematics
% Robot Modeling and Control 
% Spong, Hutchinson, Vidyasagar
% 2006

% INPUTS:
% a       :   translation  : along : x_{i}   : from : z_{i-1} : to : z_{i}
% alpha   :      rotation  : about : x_{i}   : from : z_{i-1} : to : z_{i}
% d       :   translation  : along : z_{i-1} : from : x_{i-1} : to : x_{i}
% theta   :      rotation  : about : z_{i-1} : from : x_{i-1} : to : x_{i}
% NOTE: Standard DH Parameters

% OUTPUTS:
% T       : transformation                   : from :     {i} : to : {i-1}

%%
% Rotation Transformation about z axis by theta
T_R_z = [cos(theta) -sin(theta) 0 0;
         sin(theta)  cos(theta) 0 0;
                  0           0 1 0;
                  0           0 0 1];
     
% Translation Transformation along z axis by d
T_T_z = [1 0 0 0;
         0 1 0 0;
         0 0 1 d;
         0 0 0 1];

% Translation Transformation along x axis by a
T_T_x = [1 0 0 a;
         0 1 0 0;
         0 0 1 0;
         0 0 0 1];

% Rotation Transformation about x axis by alpha
T_R_x = [1          0           0 0;
         0 cos(alpha) -sin(alpha) 0;
         0 sin(alpha)  cos(alpha) 0;
         0          0           0 1];

% For a transformation FROM frame {i} TO frame {i-1}: A
T = T_R_z*T_T_z*T_T_x*T_R_x;

end
